simulink model "rosManipCartesianTrajectory"  (R2019a)
settings: Solver=FixedStepAuto  StartTime=0.0  StopTime=inf  RelTol=1e-3
PreLoadFcn:
  | createWaypointData;
undefined symbols (not defined in the file): gen3, ts
libraries: trajExampleUtils x5, robotcorelib x2, robotlib x2, robotmaniplib x1
settings Model: Creator=scastro  LastModifiedBy=scastro
settings DataIOCC: ReturnWorkspaceOutputs=off
settings OptimizationCC: DefaultParameterBehavior=Inlined  EnhancedBackFolding=on  PassReuseOutputArgsAs=Individual arguments  OptimizeBlockOrder=speed  DifferentSizesBufferReuse=on  OptimizationCustomize=off
settings DebuggingCC: ParameterTunabilityLossMsg=error  ArithmeticOperatorsInVariantConditions=warning
settings SFSimCC: MATLABDynamicMemAlloc=off
settings RTWCC: SystemTargetFile=ert.tlc  TemplateMakefile=ert_default_tmf  GenerateReport=on  IncludeHyperlinkInReport=on  LaunchReport=on  GenerateTraceInfo=on  GenerateTraceReport=on  GenerateTraceReportSl=on  GenerateTraceReportSf=on  GenerateTraceReportEml=on
settings CodeAppCC: ForceParamTrailComments=on  IgnoreCustomStorageClasses=off  OperatorAnnotations=on  SimulinkDataObjDesc=on  SFDataObjDesc=on  InsertBlockDesc=on
settings ERTTargetCC: TargetLangStandard=C99 (ISO)  GenerateSampleERTMain=on  SupportVariableSizeSignals=on  InlinedParameterPlacement=NonHierarchical  ERTCustomFileTemplate=example_file_process.tlc

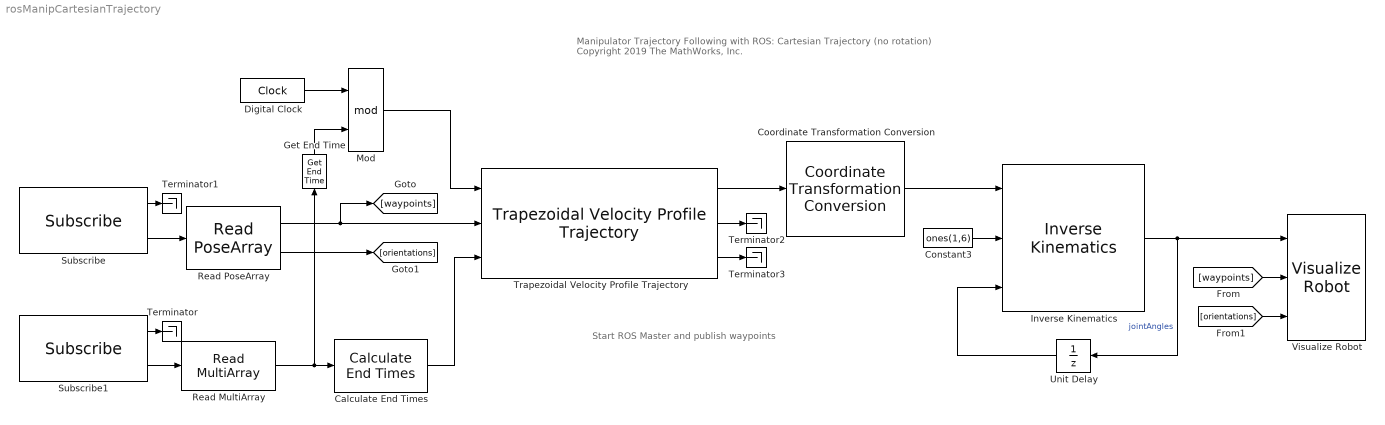
== system rosManipCartesianTrajectory ==
  note: Manipulator Trajectory Following with ROS:
      | Cartesian Trajectory (no rotation)
      |
      | Copyright 2019 The MathWorks, Inc.
  note: Start ROS Master and publish waypoints
  Calculate End Times : trajExampleUtils/Calculate End Times  maxSize=maxWaypoints  trajDof=3
      settings: SourceProductName=Simulink  SourceProductBaseCode=SL
  Constant3 : Constant  Value=ones(1,6)  VectorParams1D=off
  Coordinate Transformation Conversion : robotcorelib/Coordinate Transformation Conversion  InputRepresentation=Translation Vector  InputEulerSequence=ZYX  ShowTrVecInputPort=on  OutputRepresentation=Homogeneous Transformation  OutputEulerSequence=ZYX  ShowTrVecOutputPort=on  SimulateUsing=Interpreted execution
      settings: SourceProductBaseCode=RO
  Digital Clock : DigitalClock  SampleTime=ts
  Get End Time : trajExampleUtils/Get End Time  maxWaypoints=maxWaypoints
      settings: SourceProductName=Simulink  SourceProductBaseCode=SL
  Inverse Kinematics : robotmaniplib/Inverse Kinematics  RigidBodyTree=gen3  EndEffector=Gripper  ShowInfo=off  SolverName=BFGS Gradient Projection  EnforceJointLimits=on  MaxIterations=1500  MaxTime=10  GradientTolerance=1e-7  SolutionTolerance=1e-6  StepTolerance=1e-14  ErrorChangeTolerance=1e-12  UseErrorDamping=on  DampingBias=0.0025  SimulateUsing=Interpreted execution
      settings: SourceProductName=Robotics System Toolbox
  Mod : Math  Operator=mod  SaturateOnIntegerOverflow=on
  Read MultiArray : trajExampleUtils/Read MultiArray  maxPts=maxWaypoints
      settings: SourceProductName=Simulink  SourceProductBaseCode=SL
  Read PoseArray : trajExampleUtils/Read PoseArray  maxLength=maxWaypoints
  Subscribe : robotlib/Subscribe  topicSource=Select from ROS network  topic=/waypoints  messageType=geometry_msgs/PoseArray  sampleTime=-1  messageQueueLength=1
      settings: SourceProductBaseCode=RO
  Subscribe1 : robotlib/Subscribe  topicSource=Select from ROS network  topic=/waypoint_times  messageType=std_msgs/Float64MultiArray  sampleTime=-1  messageQueueLength=1
      settings: SourceProductBaseCode=RO
  Terminator{,1..3} (4 alike) : Terminator
  Trapezoidal Velocity Profile Trajectory : robotcorelib/Trapezoidal Velocity Profile Trajectory  WaypointSource=External  Waypoints=[ 0, -0.5, -1; 0, 0.5, 1 ]  NumParams=1  Parameter1=End Time  Parameter2=End Time  ParameterSource=External  PeakVelocity=[ 1; 1; 1 ]  Acceleration=[ 1; 2 ]  EndTime=[ 1; 1; 1 ]  AccelTime=[ 1; 2 ]  SimulateUsing=Interpreted execution
      settings: SourceProductName=Robotics System Toolbox  SourceProductBaseCode=RO
  Unit Delay : UnitDelay  InitialCondition=ikInitGuess'  SampleTime=-1  HasFrameUpgradeWarning=on
  Visualize Robot : trajExampleUtils/Visualize Robot  rbtName=gen3  eeName=Gripper  numJoints=numel(gen3.homeConfiguration)  maxPts=maxWaypoints  plotMode=Trajectory
  wires:
  Digital Clock/1 -> Mod/1
  Coordinate Transformation Conversion/1 -> Inverse Kinematics/1
  Constant3/1 -> Inverse Kinematics/2
  Inverse Kinematics/1 -> Visualize Robot/1, Unit Delay/1  "jointAngles"
  Mod/1 -> Trapezoidal Velocity Profile Trajectory/1
  Get End Time/1 -> Mod/2
  Unit Delay/1 -> Inverse Kinematics/3
  Read PoseArray/1 -> Trapezoidal Velocity Profile Trajectory/2, [waypoints]
  Trapezoidal Velocity Profile Trajectory/1 -> Coordinate Transformation Conversion/1
  [waypoints] -> Visualize Robot/2
  Read MultiArray/1 -> Get End Time/1, Calculate End Times/1
  Trapezoidal Velocity Profile Trajectory/2 -> Terminator2/1
  Trapezoidal Velocity Profile Trajectory/3 -> Terminator3/1
  [orientations] -> Visualize Robot/3
  Subscribe/2 -> Read PoseArray/1
  Read PoseArray/2 -> [orientations]
  Subscribe1/2 -> Read MultiArray/1
  Calculate End Times/1 -> Trapezoidal Velocity Profile Trajectory/3
  Subscribe1/1 -> Terminator/1
  Subscribe/1 -> Terminator1/1
